simulink model "TRAMI_DCT_AT"  (R2018b)
settings: Solver=FixedStepDiscrete  StartTime=0.0  StopTime=88  FixedStep=10e-3  RelTol=1e-3  EnableMultiTasking=on
undefined symbols (not defined in the file): CONST_AP_GEAR_SUB_NEWTRAL, CONST_AP_IDLE_SPEED_CONT, CONST_AP_LOAD_SFT, CONST_AP_LOAD_SFT_HYS, CONST_CAR_WEIGHT, CONST_CL_NUM, CONST_F_DOWN_SYNCHRO, CONST_F_SYNCHRO, CONST_F_UP_SYNCHRO, CONST_FGR, CONST_I_FlYWHEEL, CONST_INATIA_CLANK, CONST_R_SHIFT_END_CD, CONST_R_SHIFT_END_EG, CONST_R_SHIFT_END_TD, CONST_R_SHIFT_END_UP, CONST_R_SYNCHRO_ENGAGE, CONST_R_TIRE, CONST_RATIO_TQ_REDUCTION, CONST_SKIP_SHIFT_MAX, CONST_SYN_NUM, CONST_T_SFT_END_EN, CONST_T_SFT_END_JUDGE, CONST_T_SFT_END_MAX, CONST_T_SFT_END_MIN, CONST_T_SHIFT_WAIT, CONST_T_TQ_PHASE_CD, CONST_T_TQ_PHASE_ND, CONST_T_TQ_PHASE_NR, CONST_T_TQ_PHASE_TD, CONST_T_TQ_PHASE_UP, CONST_TQ_CREEP_CONT, CONST_TQ_ENGAGE_CL_MARGIN, CONST_TQ_ENGAGE_CL_MIN, CONST_TQ_INATIA_TD_SHIFT, CONST_TQ_LOAD_SFT, CONST_TQ_LOAD_SFT_HYS, CONST_TQ_ND_ENGAGE, CONST_TQ_NR_ENGAGE, CONST_TQ_TQPHASE_MIN, CONST_V_IDLE_SPEED_CONT, Eng, FALSE, GrNP, GrRev, LoopTime, MAT_CL_ENGAGE, MAT_CL_SHARE_RATE, MAT_I_ACTUATOR, MAT_SYNCHRO_COM, MAT_T_GEAR_SUB_NEWTRAL, MAT_TRANS_MGR, MaxCL, Nm, PI, Shift_CD, Shift_ND, Shift_NR, Shift_TD, Shift_Up ... (+168)
libraries: simulink x26
(part 4 of 6)

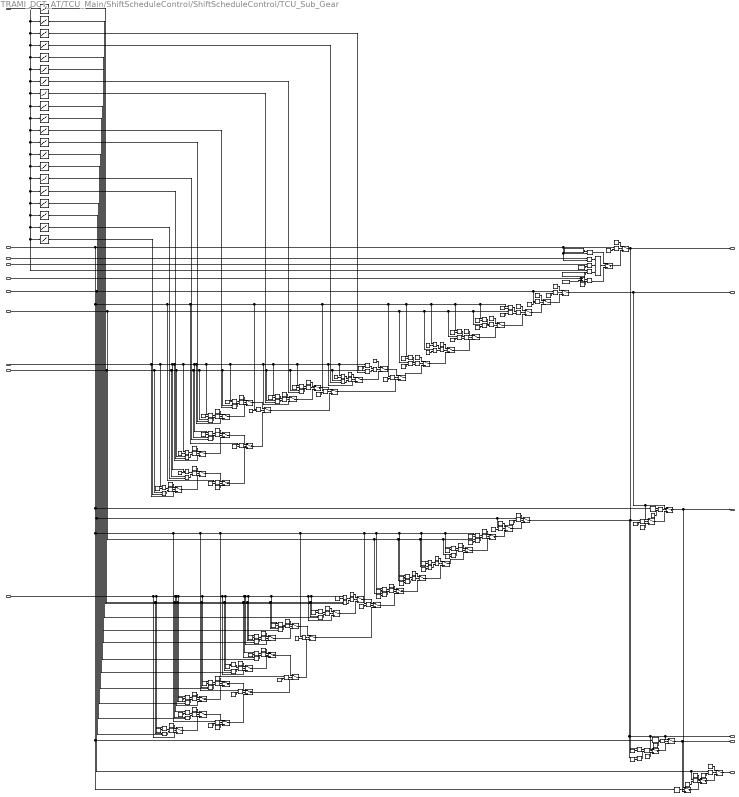
== system TRAMI_DCT_AT/TCU_Main/ShiftScheduleControl/ShiftScheduleControl/TCU_Sub_Gear ==
  accel_position : Inport  OutDataTypeStr=single
      settings: AttributesFormatString=アクセル開度[%]
  v_vehicle : Inport  Port=2  OutDataTypeStr=single
      settings: AttributesFormatString=車速[km/h]
  gear_target : Inport  Port=3  OutDataTypeStr=int16
      settings: AttributesFormatString=目標ギヤ段[-]
  gear_target_old : Inport  Port=4  OutDataTypeStr=int16
      settings: AttributesFormatString=前回の目標ギヤ段[-]
  gear_before_shift : Inport  Port=5  OutDataTypeStr=int16
      settings: AttributesFormatString=変速前ギヤ段[-]
  shifter_position : Inport  Port=6  OutDataTypeStr=int16
      settings: AttributesFormatString=|
      | シフター位置
      |  (Rev=-1; N=0 ; D=1)
      | [-]
  flag_shift : Inport  Port=7  OutDataTypeStr=boolean
      settings: AttributesFormatString=シフトフラグ[-]
  t_neutral_old : Inport  Port=8  OutDataTypeStr=single
      settings: AttributesFormatString=前回のニュートラル移行時間[ms]
  gear_sub1_tmp_old : Inport  Port=9  OutDataTypeStr=int16
      settings: AttributesFormatString=前回の待機ギヤ段（奇数軸）用中間データ[-]
  gear_sub2_tmp_old : Inport  Port=10  OutDataTypeStr=int16
      settings: AttributesFormatString=前回の待機ギヤ段（偶数軸）用中間データ[-]
  Add : Sum  Inputs=+-  OutDataTypeStr=single
  Bitwise Operator : simulink/Logic and Bit Operations/Bitwise Operator  logicop=AND  UseBitMask=on  BitMask=hex2dec('01')  BitMaskRealWorld=Stored Integer
  Bitwise Operator1 : simulink/Logic and Bit Operations/Bitwise Operator  logicop=AND  UseBitMask=on  BitMask=hex2dec('01')  BitMaskRealWorld=Stored Integer
  Bitwise Operator2 : simulink/Logic and Bit Operations/Bitwise Operator  logicop=AND  UseBitMask=on  BitMask=hex2dec('01')  BitMaskRealWorld=Stored Integer
  Constant : Constant  Value=GrRev  OutDataTypeStr=int16
  Constant1 : Constant  Value=0.0  OutDataTypeStr=single
  Constant10 : Constant  Value=0.0  OutDataTypeStr=single
  Constant{46,61,65,70,96..97,100..101} (8 alike) : Constant  Value=5  OutDataTypeStr=int16
  Constant{6,12..14,31,33,36,64,67,69,81,85,92,99,102,107,112} (17 alike) : Constant  Value=0  OutDataTypeStr=int16
  Constant{53,71..73,103..106} (8 alike) : Constant  Value=3  OutDataTypeStr=int16
  Constant{60,66,74..76,108..109} (7 alike) : Constant  OutDataTypeStr=int16
  Constant11 : Constant  Value=-1  OutDataTypeStr=int16
  Constant{27..29,57,59,62..63,110} (8 alike) : Constant  Value=2  OutDataTypeStr=int16
  Constant{15..17,34..35,77,79,88} (8 alike) : Constant  Value=10  OutDataTypeStr=int16
  Constant{18..20,37..38,41..42,82,84} (9 alike) : Constant  Value=8  OutDataTypeStr=int16
  Constant2 : Constant  Value=TRUE  OutDataTypeStr=boolean
  Constant{21..23,43,45,48..49,91} (8 alike) : Constant  Value=6  OutDataTypeStr=int16
  Constant{24..26,50,52,55..56,98} (8 alike) : Constant  Value=4  OutDataTypeStr=int16
  Constant{30,40,44,47,83,86..87} (7 alike) : Constant  Value=9  OutDataTypeStr=int16
  Constant{39,51,54,58,89..90,93..94} (8 alike) : Constant  Value=7  OutDataTypeStr=int16
  Constant5 : Constant  Value=-1  OutDataTypeStr=int16
  Constant68 : Constant  Value=0.0  OutDataTypeStr=single
  Constant7 : Constant  Value=CONST_AP_GEAR_SUB_NEWTRAL  OutDataTypeStr=int16
  Constant8 : Constant  Value=MAT_T_GEAR_SUB_NEWTRAL  OutDataTypeStr=int16
  Constant80 : Constant  Value=11  OutDataTypeStr=int16
  Constant9 : Constant  Value=LoopTime  OutDataTypeStr=single
  Constant95 : Constant  Value=-1  OutDataTypeStr=int16
  Logical Operator : Logic  Operator=OR  Inputs=3  AllPortsSameDT=off  OutDataTypeStr=boolean
  Logical Operator{1..15,17..31} (30 alike) : Logic  Operator=OR  AllPortsSameDT=off  OutDataTypeStr=boolean
  Logical Operator33 : Logic  AllPortsSameDT=off  OutDataTypeStr=boolean
  MinMax : MinMax  Function=max  Inputs=2  OutDataTypeStr=single
  Relational Operator{,2,6..18,23,28,33,38,43,45..57,62,67,72,77,85..86} (39 alike) : RelationalOperator  Operator===  OutDataTypeStr=boolean  RndMeth=Nearest
  Relational Operator1 : RelationalOperator  Operator=~=  OutDataTypeStr=boolean  RndMeth=Nearest
  Relational Operator{19,24,29,34,39,44,58,63,68,73,78,82..83} (13 alike) : RelationalOperator  Operator=>  OutDataTypeStr=boolean  RndMeth=Nearest
  Relational Operator{20,25,30,35,40,59,64,69,74,79} (10 alike) : RelationalOperator  OutDataTypeStr=boolean  RndMeth=Nearest
  Relational Operator{5,21..22,26..27,31..32,36..37,41..42,60..61,65..66,70..71,75..76,80..81} (21 alike) : RelationalOperator  Operator=<  OutDataTypeStr=boolean  RndMeth=Nearest
  Relational Operator84 : RelationalOperator  Operator=<=  OutDataTypeStr=boolean  RndMeth=Nearest
  Selector : Selector  IndexMode=Zero-based  InputPortWidth=11  IndexOptions=Index vector (port)  Indices=[1 3]  OutputSizes=1
  Switch : Switch  Criteria=u2 > Threshold  OutDataTypeStr=single
  Switch1 : Switch  Criteria=u2 > Threshold  OutDataTypeStr=single
  Switch{2..52} (51 alike) : Switch  Criteria=u2 > Threshold  OutDataTypeStr=int16
  Table_search_2D1 : Lookup_n-D  NumberOfTableDimensions=1  BreakpointsForDimension1=T2D_V_SGR_10D_X  Table=T2D_V_SGR_10D_Y  TableDataTypeStr=single  ExtrapMethod=Clip  UseLastTableValue=on  InternalRulePriority=Speed  OutDataTypeStr=single  RndMeth=Simplest  InputSameDT=on
      settings: AttributesFormatString=|
      | tbl = %<Table>
      | axis = %<BreakpointsForDimension1>
  Table_search_2D10 : Lookup_n-D  NumberOfTableDimensions=1  BreakpointsForDimension1=T2D_V_SGR_8D_X  Table=T2D_V_SGR_8D_Y  TableDataTypeStr=single  ExtrapMethod=Clip  UseLastTableValue=on  InternalRulePriority=Speed  OutDataTypeStr=single  RndMeth=Simplest  InputSameDT=on
      settings: AttributesFormatString=|
      | tbl = %<Table>
      | axis = %<BreakpointsForDimension1>
  Table_search_2D11 : Lookup_n-D  NumberOfTableDimensions=1  BreakpointsForDimension1=T2D_V_SGR_5D_X  Table=T2D_V_SGR_5D_Y  TableDataTypeStr=single  ExtrapMethod=Clip  UseLastTableValue=on  InternalRulePriority=Speed  OutDataTypeStr=single  RndMeth=Simplest  InputSameDT=on
      settings: AttributesFormatString=|
      | tbl = %<Table>
      | axis = %<BreakpointsForDimension1>
  Table_search_2D12 : Lookup_n-D  NumberOfTableDimensions=1  BreakpointsForDimension1=T2D_V_SGR_3D_X  Table=T2D_V_SGR_3D_Y  TableDataTypeStr=single  ExtrapMethod=Clip  UseLastTableValue=on  InternalRulePriority=Speed  OutDataTypeStr=single  RndMeth=Simplest  InputSameDT=on
      settings: AttributesFormatString=|
      | tbl = %<Table>
      | axis = %<BreakpointsForDimension1>
  Table_search_2D13 : Lookup_n-D  NumberOfTableDimensions=1  BreakpointsForDimension1=T2D_V_SGR_4U_X  Table=T2D_V_SGR_4U_Y  TableDataTypeStr=single  ExtrapMethod=Clip  UseLastTableValue=on  InternalRulePriority=Speed  OutDataTypeStr=single  RndMeth=Simplest  InputSameDT=on
      settings: AttributesFormatString=|
      | tbl = %<Table>
      | axis = %<BreakpointsForDimension1>
  Table_search_2D14 : Lookup_n-D  NumberOfTableDimensions=1  BreakpointsForDimension1=T2D_V_SGR_4D_X  Table=T2D_V_SGR_4D_Y  TableDataTypeStr=single  ExtrapMethod=Clip  UseLastTableValue=on  InternalRulePriority=Speed  OutDataTypeStr=single  RndMeth=Simplest  InputSameDT=on
      settings: AttributesFormatString=|
      | tbl = %<Table>
      | axis = %<BreakpointsForDimension1>
  Table_search_2D15 : Lookup_n-D  NumberOfTableDimensions=1  BreakpointsForDimension1=T2D_V_SGR_3U_X  Table=T2D_V_SGR_3U_Y  TableDataTypeStr=single  ExtrapMethod=Clip  UseLastTableValue=on  InternalRulePriority=Speed  OutDataTypeStr=single  RndMeth=Simplest  InputSameDT=on
      settings: AttributesFormatString=|
      | tbl = %<Table>
      | axis = %<BreakpointsForDimension1>
  Table_search_2D16 : Lookup_n-D  NumberOfTableDimensions=1  BreakpointsForDimension1=T2D_V_SGR_2U_X  Table=T2D_V_SGR_2U_Y  TableDataTypeStr=single  ExtrapMethod=Clip  UseLastTableValue=on  InternalRulePriority=Speed  OutDataTypeStr=single  RndMeth=Simplest  InputSameDT=on
      settings: AttributesFormatString=|
      | tbl = %<Table>
      | axis = %<BreakpointsForDimension1>
  Table_search_2D17 : Lookup_n-D  NumberOfTableDimensions=1  BreakpointsForDimension1=T2D_V_SGR_5U_X  Table=T2D_V_SGR_5U_Y  TableDataTypeStr=single  ExtrapMethod=Clip  UseLastTableValue=on  InternalRulePriority=Speed  OutDataTypeStr=single  RndMeth=Simplest  InputSameDT=on
      settings: AttributesFormatString=|
      | tbl = %<Table>
      | axis = %<BreakpointsForDimension1>
  Table_search_2D18 : Lookup_n-D  NumberOfTableDimensions=1  BreakpointsForDimension1=T2D_V_SGR_2D_X  Table=T2D_V_SGR_2D_Y  TableDataTypeStr=single  ExtrapMethod=Clip  UseLastTableValue=on  InternalRulePriority=Speed  OutDataTypeStr=single  RndMeth=Simplest  InputSameDT=on
      settings: AttributesFormatString=|
      | tbl = %<Table>
      | axis = %<BreakpointsForDimension1>
  Table_search_2D19 : Lookup_n-D  NumberOfTableDimensions=1  BreakpointsForDimension1=T2D_V_SGR_1U_X  Table=T2D_V_SGR_1U_Y  TableDataTypeStr=single  ExtrapMethod=Clip  UseLastTableValue=on  InternalRulePriority=Speed  OutDataTypeStr=single  RndMeth=Simplest  InputSameDT=on
      settings: AttributesFormatString=|
      | tbl = %<Table>
      | axis = %<BreakpointsForDimension1>
  Table_search_2D2 : Lookup_n-D  NumberOfTableDimensions=1  BreakpointsForDimension1=T2D_V_SGR_9U_X  Table=T2D_V_SGR_9U_Y  TableDataTypeStr=single  ExtrapMethod=Clip  UseLastTableValue=on  InternalRulePriority=Speed  OutDataTypeStr=single  RndMeth=Simplest  InputSameDT=on
      settings: AttributesFormatString=|
      | tbl = %<Table>
      | axis = %<BreakpointsForDimension1>
  Table_search_2D20 : Lookup_n-D  NumberOfTableDimensions=1  BreakpointsForDimension1=T2D_V_SGR_1D_X  Table=T2D_V_SGR_1D_Y  TableDataTypeStr=single  ExtrapMethod=Clip  UseLastTableValue=on  InternalRulePriority=Speed  OutDataTypeStr=single  RndMeth=Simplest  InputSameDT=on
      settings: AttributesFormatString=|
      | tbl = %<Table>
      | axis = %<BreakpointsForDimension1>
  Table_search_2D3 : Lookup_n-D  NumberOfTableDimensions=1  BreakpointsForDimension1=T2D_V_SGR_9D_X  Table=T2D_V_SGR_9D_Y  TableDataTypeStr=single  ExtrapMethod=Clip  UseLastTableValue=on  InternalRulePriority=Speed  OutDataTypeStr=single  RndMeth=Simplest  InputSameDT=on
      settings: AttributesFormatString=|
      | tbl = %<Table>
      | axis = %<BreakpointsForDimension1>
  Table_search_2D4 : Lookup_n-D  NumberOfTableDimensions=1  BreakpointsForDimension1=T2D_V_SGR_8U_X  Table=T2D_V_SGR_8U_Y  TableDataTypeStr=single  ExtrapMethod=Clip  UseLastTableValue=on  InternalRulePriority=Speed  OutDataTypeStr=single  RndMeth=Simplest  InputSameDT=on
      settings: AttributesFormatString=|
      | tbl = %<Table>
      | axis = %<BreakpointsForDimension1>
  Table_search_2D5 : Lookup_n-D  NumberOfTableDimensions=1  BreakpointsForDimension1=T2D_V_SGR_7U_X  Table=T2D_V_SGR_7U_Y  TableDataTypeStr=single  ExtrapMethod=Clip  UseLastTableValue=on  InternalRulePriority=Speed  OutDataTypeStr=single  RndMeth=Simplest  InputSameDT=on
      settings: AttributesFormatString=|
      | tbl = %<Table>
      | axis = %<BreakpointsForDimension1>
  Table_search_2D6 : Lookup_n-D  NumberOfTableDimensions=1  BreakpointsForDimension1=T2D_V_SGR_10U_X  Table=T2D_V_SGR_10U_Y  TableDataTypeStr=single  ExtrapMethod=Clip  UseLastTableValue=on  InternalRulePriority=Speed  OutDataTypeStr=single  RndMeth=Simplest  InputSameDT=on
      settings: AttributesFormatString=|
      | tbl = %<Table>
      | axis = %<BreakpointsForDimension1>
  Table_search_2D7 : Lookup_n-D  NumberOfTableDimensions=1  BreakpointsForDimension1=T2D_V_SGR_7D_X  Table=T2D_V_SGR_7D_Y  TableDataTypeStr=single  ExtrapMethod=Clip  UseLastTableValue=on  InternalRulePriority=Speed  OutDataTypeStr=single  RndMeth=Simplest  InputSameDT=on
      settings: AttributesFormatString=|
      | tbl = %<Table>
      | axis = %<BreakpointsForDimension1>
  Table_search_2D8 : Lookup_n-D  NumberOfTableDimensions=1  BreakpointsForDimension1=T2D_V_SGR_6U_X  Table=T2D_V_SGR_6U_Y  TableDataTypeStr=single  ExtrapMethod=Clip  UseLastTableValue=on  InternalRulePriority=Speed  OutDataTypeStr=single  RndMeth=Simplest  InputSameDT=on
      settings: AttributesFormatString=|
      | tbl = %<Table>
      | axis = %<BreakpointsForDimension1>
  Table_search_2D9 : Lookup_n-D  NumberOfTableDimensions=1  BreakpointsForDimension1=T2D_V_SGR_6D_X  Table=T2D_V_SGR_6D_Y  TableDataTypeStr=single  ExtrapMethod=Clip  UseLastTableValue=on  InternalRulePriority=Speed  OutDataTypeStr=single  RndMeth=Simplest  InputSameDT=on
      settings: AttributesFormatString=|
      | tbl = %<Table>
      | axis = %<BreakpointsForDimension1>
  gear_sub : Outport  OutDataTypeStr=int16  PortDimensions=1
      settings: AttributesFormatString=待機ギヤ段[-]
  gear_sub1 : Outport  Port=2  OutDataTypeStr=int16  PortDimensions=1
      settings: AttributesFormatString=待機ギヤ段（奇数軸）
  gear_sub2 : Outport  Port=3  OutDataTypeStr=int16  PortDimensions=1
      settings: AttributesFormatString=待機ギヤ段（偶数軸）[-]
  t_neutral : Outport  Port=4  OutDataTypeStr=single  PortDimensions=1
      settings: AttributesFormatString=ニュートラル移行時間[ms]
  gear_sub1_tmp : Outport  Port=5  OutDataTypeStr=int16  PortDimensions=1
      settings: AttributesFormatString=待機ギヤ段（奇数軸）用中間データ[-]
  gear_sub2_tmp : Outport  Port=6  OutDataTypeStr=int16  PortDimensions=1
      settings: AttributesFormatString=待機ギヤ段（偶数軸）用中間データ[-]
  wires:
  accel_position/1 -> Table_search_2D5/1, Table_search_2D20/1, Relational Operator5/1, Table_search_2D19/1, Table_search_2D18/1, Table_search_2D16/1, Table_search_2D12/1, Table_search_2D15/1, Table_search_2D14/1, Table_search_2D13/1, Table_search_2D11/1, Table_search_2D17/1, Table_search_2D9/1, Table_search_2D8/1, Table_search_2D7/1, Table_search_2D10/1, Table_search_2D4/1, Table_search_2D3/1, Table_search_2D2/1, Table_search_2D1/1, Table_search_2D6/1  "accel_position"
  Relational Operator/1 -> Switch/2
  Constant1/1 -> Switch/1
  Switch1/1 -> Switch/3
  Switch/1 -> t_neutral/1, Relational Operator44/1, Relational Operator83/1  "t_neutral"
  gear_target_old/1 -> Relational Operator1/1  "gear_target_old"
  flag_shift/1 -> Relational Operator2/1  "flag_shift"
  Constant/1 -> Relational Operator/2
  Constant2/1 -> Relational Operator2/2
  gear_sub1_tmp_old/1 -> Relational Operator68/1, Relational Operator58/1, Relational Operator60/1, Switch35/3, Relational Operator63/1, Relational Operator65/1, Switch38/3, Relational Operator70/1, Switch41/3, Relational Operator73/1, Relational Operator75/1, Switch44/3, Relational Operator78/1, Relational Operator80/1, Switch47/3
  Relational Operator1/1 -> Logical Operator/1
  Relational Operator2/1 -> Logical Operator/2
  Constant7/1 -> Relational Operator5/2
  Relational Operator5/1 -> Logical Operator/3
  Logical Operator/1 -> Switch1/2
  Selector/1 -> Switch1/1
  Constant8/1 -> Selector/1
  MinMax/1 -> Switch1/3
  Add/1 -> MinMax/1
  Constant9/1 -> Add/2
  Constant10/1 -> MinMax/2
  t_neutral_old/1 -> Add/1
  Relational Operator6/1 -> Switch2/2
  Constant11/1 -> Relational Operator6/2
  Constant12/1 -> Switch2/1
  Switch3/1 -> Switch2/3
  Relational Operator7/1 -> Switch3/2
  Constant13/1 -> Relational Operator7/2
  Constant14/1 -> Switch3/1
  Switch4/1 -> Switch3/3
  Logical Operator1/1 -> Switch4/2
  Constant15/1 -> Switch4/1
  Relational Operator9/1 -> Logical Operator1/2
  Relational Operator8/1 -> Logical Operator1/1
  Constant16/1 -> Relational Operator8/2
  Constant17/1 -> Relational Operator9/2
  Switch5/1 -> Switch4/3
  Switch6/1 -> Switch5/3
  Constant20/1 -> Relational Operator11/2
  Constant19/1 -> Relational Operator10/2
  Relational Operator10/1 -> Logical Operator2/1
  Relational Operator11/1 -> Logical Operator2/2
  Constant18/1 -> Switch5/1
  Logical Operator2/1 -> Switch5/2
  Logical Operator3/1 -> Switch6/2
  Constant21/1 -> Switch6/1
  Relational Operator13/1 -> Logical Operator3/2
  Relational Operator12/1 -> Logical Operator3/1
  Constant22/1 -> Relational Operator12/2
  Constant23/1 -> Relational Operator13/2
  Switch7/1 -> Switch6/3
  Switch8/1 -> Switch7/3
  Constant26/1 -> Relational Operator15/2
  Constant25/1 -> Relational Operator14/2
  Relational Operator14/1 -> Logical Operator4/1
  Relational Operator15/1 -> Logical Operator4/2
  Constant24/1 -> Switch7/1
  Logical Operator4/1 -> Switch7/2
  Logical Operator5/1 -> Switch8/2
  Constant27/1 -> Switch8/1
  Relational Operator17/1 -> Logical Operator5/2
  Relational Operator16/1 -> Logical Operator5/1
  Constant28/1 -> Relational Operator16/2
  Constant29/1 -> Relational Operator17/2
  Switch9/1 -> Switch8/3
  Relational Operator18/1 -> Switch9/2
  Constant30/1 -> Relational Operator18/2
  Switch10/1 -> Switch9/1
  gear_sub2_tmp_old/1 -> Relational Operator41/1, Relational Operator39/1, Relational Operator36/1, Relational Operator34/1, Relational Operator31/1, Relational Operator29/1, Relational Operator24/1, Relational Operator19/1, Relational Operator21/1, Switch11/3, Relational Operator26/1, Switch14/3, Switch17/3, Switch20/3, Switch23/3  "gear_sub2_tmp"
  Constant34/1 -> Relational Operator19/2
  Logical Operator6/1 -> Switch10/2
  Relational Operator19/1 -> Logical Operator6/1
  Relational Operator20/1 -> Logical Operator6/2
  Table_search_2D2/1 -> Relational Operator20/2  "ans"
  Constant35/1 -> Switch10/1
  Switch11/1 -> Switch10/3
  Constant38/1 -> Switch11/1
  Table_search_2D3/1 -> Relational Operator22/2  "ans"
  Relational Operator22/1 -> Logical Operator7/2
  Relational Operator21/1 -> Logical Operator7/1
  Logical Operator7/1 -> Switch11/2
  Constant37/1 -> Relational Operator21/2
  Switch2/1 -> gear_sub2_tmp/1, Switch25/1, Switch24/1  "gear_sub2_tmp"
  Relational Operator23/1 -> Switch12/2
  Constant39/1 -> Relational Operator23/2
  Switch13/1 -> Switch12/1
  Logical Operator8/1 -> Switch13/2
  Relational Operator24/1 -> Logical Operator8/1
  Constant41/1 -> Relational Operator24/2
  Relational Operator25/1 -> Logical Operator8/2
  Table_search_2D5/1 -> Relational Operator25/2  "ans"
  Constant42/1 -> Switch13/1
  Switch14/1 -> Switch13/3
  Relational Operator27/1 -> Logical Operator9/2
  Relational Operator26/1 -> Logical Operator9/1
  Logical Operator9/1 -> Switch14/2
  Constant43/1 -> Switch14/1
  Constant45/1 -> Relational Operator26/2
  Table_search_2D7/1 -> Relational Operator27/2  "v_shift_sub_7dans"
  Switch15/1 -> Switch12/3
  Switch18/1 -> Switch15/3
  Table_search_2D11/1 -> Relational Operator32/2  "v_shift_sub_7dans"
  Constant52/1 -> Relational Operator31/2
  Constant50/1 -> Switch17/1
  Logical Operator11/1 -> Switch17/2
  Relational Operator31/1 -> Logical Operator11/1
  Relational Operator32/1 -> Logical Operator11/2
  Switch17/1 -> Switch16/3
  Constant49/1 -> Switch16/1
  Table_search_2D17/1 -> Relational Operator30/2  "ans"
  Relational Operator30/1 -> Logical Operator10/2
  Constant48/1 -> Relational Operator29/2
  Relational Operator29/1 -> Logical Operator10/1
  Logical Operator10/1 -> Switch16/2
  Switch16/1 -> Switch15/1
  Constant46/1 -> Relational Operator28/2
  Relational Operator28/1 -> Switch15/2
  Table_search_2D15/1 -> Relational Operator35/2  "v_vehicle"
  Relational Operator33/1 -> Switch18/2
  Constant53/1 -> Relational Operator33/2
  Switch19/1 -> Switch18/1
  Logical Operator12/1 -> Switch19/2
  Relational Operator34/1 -> Logical Operator12/1
  Constant55/1 -> Relational Operator34/2
  Relational Operator35/1 -> Logical Operator12/2
  Constant56/1 -> Switch19/1
  Switch20/1 -> Switch19/3
  Relational Operator37/1 -> Logical Operator13/2
  Relational Operator36/1 -> Logical Operator13/1
  Logical Operator13/1 -> Switch20/2
  Constant57/1 -> Switch20/1
  Constant59/1 -> Relational Operator36/2
  Table_search_2D12/1 -> Relational Operator37/2  "v_shift_sub_7dans"
  Switch21/1 -> Switch18/3
  Table_search_2D20/1 -> Relational Operator42/2  "v_shift_sub_7dans"
  Constant66/1 -> Relational Operator41/2
  Constant64/1 -> Switch23/1
  Logical Operator15/1 -> Switch23/2
  Relational Operator41/1 -> Logical Operator15/1
  Relational Operator42/1 -> Logical Operator15/2
  Switch23/1 -> Switch22/3
  Constant63/1 -> Switch22/1
  Relational Operator40/1 -> Logical Operator14/2
  Constant62/1 -> Relational Operator39/2
  Relational Operator39/1 -> Logical Operator14/1
  Logical Operator14/1 -> Switch22/2
  Switch22/1 -> Switch21/1
  Constant60/1 -> Relational Operator38/2
  Relational Operator38/1 -> Switch21/2
  Table_search_2D19/1 -> Relational Operator40/2  "v_vehicle"
  Bitwise Operator/1 -> Relational Operator43/1
  Constant67/1 -> Relational Operator43/2
  Relational Operator43/1 -> Switch24/2
  Switch25/1 -> Switch24/3
  Relational Operator44/1 -> Switch25/2
  Constant68/1 -> Relational Operator44/2
  Constant69/1 -> Switch25/3
  Constant5/1 -> Relational Operator45/2
  Relational Operator45/1 -> Switch26/2
  Switch27/1 -> Switch26/3
  Constant6/1 -> Switch26/1
  Constant36/1 -> Switch27/1
  Switch28/1 -> Switch27/3
  Relational Operator46/1 -> Switch27/2
  Constant33/1 -> Relational Operator46/2
  Switch26/1 -> Switch48/1, gear_sub1_tmp/1, Switch49/1, Relational Operator84/1  "gear_sub1_tmp"
  Constant40/1 -> Relational Operator47/2
  Relational Operator47/1 -> Logical Operator17/1
  Relational Operator48/1 -> Logical Operator17/2
  Constant44/1 -> Relational Operator48/2
  Logical Operator17/1 -> Switch28/2
  Constant47/1 -> Switch28/1
  Switch29/1 -> Switch28/3
  Logical Operator18/1 -> Switch29/2
  Constant58/1 -> Switch29/1
  Switch30/1 -> Switch29/3
  Relational Operator49/1 -> Logical Operator18/1
  Constant51/1 -> Relational Operator49/2
  Relational Operator50/1 -> Logical Operator18/2
  Constant54/1 -> Relational Operator50/2
  Constant65/1 -> Relational Operator52/2
  Relational Operator52/1 -> Logical Operator19/2
  Constant61/1 -> Relational Operator51/2
  Relational Operator51/1 -> Logical Operator19/1
  Switch31/1 -> Switch30/3
  Constant70/1 -> Switch30/1
  Logical Operator19/1 -> Switch30/2
  Logical Operator20/1 -> Switch31/2
  Constant73/1 -> Switch31/1
  Switch32/1 -> Switch31/3
  Relational Operator53/1 -> Logical Operator20/1
  Constant71/1 -> Relational Operator53/2
  Relational Operator54/1 -> Logical Operator20/2
  Constant72/1 -> Relational Operator54/2
  Constant75/1 -> Relational Operator56/2
  Relational Operator56/1 -> Logical Operator21/2
  Constant74/1 -> Relational Operator55/2
  Relational Operator55/1 -> Logical Operator21/1
  Switch33/1 -> Switch32/3
  Constant76/1 -> Switch32/1
  Logical Operator21/1 -> Switch32/2
  gear_before_shift/1 -> Relational Operator17/1, Relational Operator15/1, Relational Operator13/1, Relational Operator11/1, Relational Operator9/1, Relational Operator54/1, Relational Operator50/1, Relational Operator48/1, Relational Operator52/1, Relational Operator56/1  "gear_before_shift"
  Relational Operator57/1 -> Switch33/2
  Constant77/1 -> Relational Operator57/2
  Relational Operator58/1 -> Logical Operator22/1
  Constant79/1 -> Relational Operator58/2
  Relational Operator59/1 -> Logical Operator22/2
  Table_search_2D6/1 -> Relational Operator59/2  "ans"
  Switch34/1 -> Switch33/1
  Logical Operator22/1 -> Switch34/2
  Constant80/1 -> Switch34/1
  Switch36/1 -> Switch33/3
  Constant83/1 -> Switch35/1
  Logical Operator23/1 -> Switch35/2
  Table_search_2D1/1 -> Relational Operator61/2  "ans"
  Relational Operator61/1 -> Logical Operator23/2
  Constant82/1 -> Relational Operator60/2
  Relational Operator60/1 -> Logical Operator23/1
  Switch35/1 -> Switch34/3
  Switch38/1 -> Switch37/3
  Relational Operator65/1 -> Logical Operator25/1
  Constant89/1 -> Relational Operator65/2
  Relational Operator66/1 -> Logical Operator25/2
  Table_search_2D10/1 -> Relational Operator66/2  "ans"
  Logical Operator25/1 -> Switch38/2
  Constant90/1 -> Switch38/1
  Switch39/1 -> Switch36/3
  Constant87/1 -> Switch37/1
  Logical Operator24/1 -> Switch37/2
  Switch37/1 -> Switch36/1
  Table_search_2D4/1 -> Relational Operator64/2  "ans"
  Relational Operator64/1 -> Logical Operator24/2
  Constant86/1 -> Relational Operator63/2
  Relational Operator63/1 -> Logical Operator24/1
  Constant84/1 -> Relational Operator62/2
  Relational Operator62/1 -> Switch36/2
  Relational Operator67/1 -> Switch39/2
  Constant91/1 -> Relational Operator67/2
  Relational Operator68/1 -> Logical Operator26/1
  Constant93/1 -> Relational Operator68/2
  Relational Operator69/1 -> Logical Operator26/2
  Table_search_2D8/1 -> Relational Operator69/2  "ans"
  Switch40/1 -> Switch39/1
  Logical Operator26/1 -> Switch40/2
  Constant94/1 -> Switch40/1
  Switch42/1 -> Switch39/3
  Constant97/1 -> Switch41/1
  Logical Operator27/1 -> Switch41/2
  Table_search_2D9/1 -> Relational Operator71/2  "ans"
  Relational Operator71/1 -> Logical Operator27/2
  Constant96/1 -> Relational Operator70/2
  Relational Operator70/1 -> Logical Operator27/1
  Switch41/1 -> Switch40/3
  Switch44/1 -> Switch43/3
  Relational Operator75/1 -> Logical Operator29/1
  Constant103/1 -> Relational Operator75/2
  Relational Operator76/1 -> Logical Operator29/2
  Table_search_2D14/1 -> Relational Operator76/2  "ans"
  Logical Operator29/1 -> Switch44/2
  Constant104/1 -> Switch44/1
  Switch45/1 -> Switch42/3
  Constant101/1 -> Switch43/1
  Logical Operator28/1 -> Switch43/2
  Switch43/1 -> Switch42/1
  Table_search_2D13/1 -> Relational Operator74/2  "ans"
  Relational Operator74/1 -> Logical Operator28/2
  Constant100/1 -> Relational Operator73/2
  Relational Operator73/1 -> Logical Operator28/1
  Constant98/1 -> Relational Operator72/2
  Relational Operator72/1 -> Switch42/2
  v_vehicle/1 -> Relational Operator40/1, Relational Operator37/1, Relational Operator35/1, Relational Operator32/1, Relational Operator30/1, Relational Operator27/1, Relational Operator22/1, Relational Operator20/1, Relational Operator25/1, Relational Operator42/1, Relational Operator81/1, Relational Operator79/1, Relational Operator76/1, Relational Operator74/1, Relational Operator71/1, Relational Operator69/1, Relational Operator66/1, Relational Operator61/1, Relational Operator59/1, Relational Operator64/1  "v_vehicle"
  Relational Operator77/1 -> Switch45/2
  Constant110/1 -> Relational Operator77/2
  Relational Operator78/1 -> Logical Operator30/1
  Constant105/1 -> Relational Operator78/2
  Relational Operator79/1 -> Logical Operator30/2
  Table_search_2D16/1 -> Relational Operator79/2  "ans"
  Switch46/1 -> Switch45/1
  Logical Operator30/1 -> Switch46/2
  Constant106/1 -> Switch46/1
  Constant112/1 -> Switch45/3
  Constant109/1 -> Switch47/1
  Logical Operator31/1 -> Switch47/2
  Table_search_2D18/1 -> Relational Operator81/2  "ans"
  Relational Operator81/1 -> Logical Operator31/2
  Constant108/1 -> Relational Operator80/2
  Relational Operator80/1 -> Logical Operator31/1
  Switch47/1 -> Switch46/3
  gear_target/1 -> Relational Operator1/2, Selector/2, Relational Operator/1, Relational Operator8/1, Relational Operator10/1, Relational Operator12/1, Relational Operator14/1, Relational Operator16/1, Relational Operator18/1, Relational Operator23/1, Relational Operator28/1, Relational Operator33/1, Relational Operator38/1, Bitwise Operator/1, Relational Operator77/1, Relational Operator47/1, Relational Operator49/1, Relational Operator51/1, Relational Operator53/1, Relational Operator55/1, Relational Operator57/1, Relational Operator62/1, Relational Operator67/1, Relational Operator72/1, Bitwise Operator1/1, Bitwise Operator2/1
  Bitwise Operator1/1 -> Relational Operator82/1
  Constant81/1 -> Relational Operator82/2
  Relational Operator82/1 -> Switch48/2
  Switch48/1 -> gear_sub1/1, Switch52/3  "gear_sub1"
  Constant85/1 -> Relational Operator83/2
  Relational Operator83/1 -> Logical Operator33/1
  Relational Operator84/1 -> Logical Operator33/2
  Constant88/1 -> Relational Operator84/2
  Logical Operator33/1 -> Switch49/2
  Switch49/1 -> Switch48/3  "gear_sub1"
  Constant92/1 -> Switch49/3
  Relational Operator85/1 -> Switch50/2
  Constant102/1 -> Switch50/1
  Switch51/1 -> Switch50/3
  shifter_position/1 -> Relational Operator6/1, Relational Operator7/1, Relational Operator46/1, Relational Operator45/1, Relational Operator86/1, Relational Operator85/1  "shifter_position"
  Constant95/1 -> Relational Operator85/2
  Constant99/1 -> Relational Operator86/2
  Switch52/1 -> Switch51/3
  Constant107/1 -> Switch51/1
  Relational Operator86/1 -> Switch51/2
  Bitwise Operator2/1 -> Switch52/2
  Switch50/1 -> gear_sub/1  "gear_sub"
  Switch24/1 -> gear_sub2/1, Switch52/1  "gear_sub2"
  Constant31/1 -> Switch21/3
  Switch12/1 -> Switch9/3

== system TRAMI_DCT_AT/TCU_Main/ShiftScheduleControl/ShiftScheduleControl/TCU_Tsp_Each_Gear ==
  r_gearbox_output : Inport  OutDataTypeStr=single
      settings: AttributesFormatString=GearBox出力回転[rpm]
  Gain : Gain  Gain=MAT_TRANS_MGR  OutDataTypeStr=single
  r_gb_input_each_gear : Outport  OutDataTypeStr=single
      settings: AttributesFormatString=|
      | 各ギヤ段でのGearBox入力回転
      | 配列数12: 左から N, 1st, 2nd, 3rd ,4th ,5th ,6th ,7th, 8th, 9th, 10th, Rev[rpm]
  wires:
  r_gearbox_output/1 -> Gain/1
  Gain/1 -> r_gb_input_each_gear/1  "r_gb_input_each_gear"

== system TRAMI_DCT_AT/TCU_Main/ShiftScheduleControl/ShiftScheduleControl/cUnitDelay1 ==
  <param> : Inport
  Constant13 : Constant  Value=initParam  OutDataTypeStr=int16
  Switch12 : Switch  Criteria=u2 > Threshold
  Unit Delay2 : UnitDelay  InitialCondition=zeros(size(initParam))  SampleTime=-1
  preParam : Outport
  wires:
  <param>/1 -> Unit Delay2/1
  Constant13/1 -> Switch12/1
  [FlagInit] -> Switch12/2
  Switch12/1 -> preParam/1
  Unit Delay2/1 -> Switch12/3

== system TRAMI_DCT_AT/TCU_Main/ShiftScheduleControl/ShiftScheduleControl/cUnitDelay10 ==
  <param> : Inport
  Constant13 : Constant  Value=initParam  OutDataTypeStr=single
  Switch12 : Switch  Criteria=u2 > Threshold
  Unit Delay2 : UnitDelay  InitialCondition=zeros(size(initParam))  SampleTime=-1
  preParam : Outport
  wires:
  Unit Delay2/1 -> Switch12/3
  Switch12/1 -> preParam/1
  [FlagInit] -> Switch12/2
  Constant13/1 -> Switch12/1
  <param>/1 -> Unit Delay2/1

== system TRAMI_DCT_AT/TCU_Main/ShiftScheduleControl/ShiftScheduleControl/cUnitDelay11 ==
  <param> : Inport
  Constant13 : Constant  Value=initParam  OutDataTypeStr=boolean
  Switch12 : Switch  Criteria=u2 > Threshold
  Unit Delay2 : UnitDelay  InitialCondition=zeros(size(initParam))  SampleTime=-1
  preParam : Outport
  wires:
  Unit Delay2/1 -> Switch12/3
  Switch12/1 -> preParam/1
  [FlagInit] -> Switch12/2
  Constant13/1 -> Switch12/1
  <param>/1 -> Unit Delay2/1

== system TRAMI_DCT_AT/TCU_Main/ShiftScheduleControl/ShiftScheduleControl/cUnitDelay12 ==
  <param> : Inport
  Constant13 : Constant  Value=initParam  OutDataTypeStr=single
  Switch12 : Switch  Criteria=u2 > Threshold
  Unit Delay2 : UnitDelay  InitialCondition=zeros(size(initParam))  SampleTime=-1
  preParam : Outport
  wires:
  <param>/1 -> Unit Delay2/1
  Constant13/1 -> Switch12/1
  [FlagInit] -> Switch12/2
  Switch12/1 -> preParam/1
  Unit Delay2/1 -> Switch12/3

== system TRAMI_DCT_AT/TCU_Main/ShiftScheduleControl/ShiftScheduleControl/cUnitDelay13 ==
  <param> : Inport
  Constant13 : Constant  Value=initParam  OutDataTypeStr=int16
  Switch12 : Switch  Criteria=u2 > Threshold
  Unit Delay2 : UnitDelay  InitialCondition=zeros(size(initParam))  SampleTime=-1
  preParam : Outport  OutDataTypeStr=int16
  wires:
  Unit Delay2/1 -> Switch12/3
  Switch12/1 -> preParam/1
  [FlagInit] -> Switch12/2
  Constant13/1 -> Switch12/1
  <param>/1 -> Unit Delay2/1

== system TRAMI_DCT_AT/TCU_Main/ShiftScheduleControl/ShiftScheduleControl/cUnitDelay14 ==
  <param> : Inport
  Constant13 : Constant  Value=initParam  OutDataTypeStr=single
  Switch12 : Switch  Criteria=u2 > Threshold
  Unit Delay2 : UnitDelay  InitialCondition=zeros(size(initParam))  SampleTime=-1
  preParam : Outport
  wires:
  Unit Delay2/1 -> Switch12/3
  Switch12/1 -> preParam/1
  [FlagInit] -> Switch12/2
  Constant13/1 -> Switch12/1
  <param>/1 -> Unit Delay2/1

== system TRAMI_DCT_AT/TCU_Main/ShiftScheduleControl/ShiftScheduleControl/cUnitDelay15 ==
  <param> : Inport
  Constant13 : Constant  Value=initParam  OutDataTypeStr=int16
  Switch12 : Switch  Criteria=u2 > Threshold
  Unit Delay2 : UnitDelay  InitialCondition=zeros(size(initParam))  SampleTime=-1
  preParam : Outport
  wires:
  <param>/1 -> Unit Delay2/1
  Constant13/1 -> Switch12/1
  [FlagInit] -> Switch12/2
  Switch12/1 -> preParam/1
  Unit Delay2/1 -> Switch12/3

== system TRAMI_DCT_AT/TCU_Main/ShiftScheduleControl/ShiftScheduleControl/cUnitDelay2 ==
  <param> : Inport
  Constant13 : Constant  Value=initParam  OutDataTypeStr=int16
  Switch12 : Switch  Criteria=u2 > Threshold
  Unit Delay2 : UnitDelay  InitialCondition=zeros(size(initParam))  SampleTime=-1
  preParam : Outport
  wires:
  Unit Delay2/1 -> Switch12/3
  Switch12/1 -> preParam/1
  [FlagInit] -> Switch12/2
  Constant13/1 -> Switch12/1
  <param>/1 -> Unit Delay2/1

== system TRAMI_DCT_AT/TCU_Main/ShiftScheduleControl/ShiftScheduleControl/cUnitDelay3 ==
  <param> : Inport
  Constant13 : Constant  Value=initParam  OutDataTypeStr=int16
  Switch12 : Switch  Criteria=u2 > Threshold
  Unit Delay2 : UnitDelay  InitialCondition=zeros(size(initParam))  SampleTime=-1
  preParam : Outport
  wires:
  <param>/1 -> Unit Delay2/1
  Constant13/1 -> Switch12/1
  [FlagInit] -> Switch12/2
  Switch12/1 -> preParam/1
  Unit Delay2/1 -> Switch12/3

== system TRAMI_DCT_AT/TCU_Main/ShiftScheduleControl/ShiftScheduleControl/cUnitDelay4 ==
  <param> : Inport
  Constant13 : Constant  Value=initParam  OutDataTypeStr=boolean
  Switch12 : Switch  Criteria=u2 > Threshold
  Unit Delay2 : UnitDelay  InitialCondition=zeros(size(initParam))  SampleTime=-1
  preParam : Outport
  wires:
  Unit Delay2/1 -> Switch12/3
  Switch12/1 -> preParam/1
  [FlagInit] -> Switch12/2
  Constant13/1 -> Switch12/1
  <param>/1 -> Unit Delay2/1

== system TRAMI_DCT_AT/TCU_Main/ShiftScheduleControl/ShiftScheduleControl/cUnitDelay5 ==
  <param> : Inport
  Constant13 : Constant  Value=initParam  OutDataTypeStr=boolean
  Switch12 : Switch  Criteria=u2 > Threshold  OutDataTypeStr=boolean
  Unit Delay2 : UnitDelay  InitialCondition=zeros(size(initParam))  SampleTime=-1
  preParam : Outport
  wires:
  <param>/1 -> Unit Delay2/1
  Constant13/1 -> Switch12/1
  [FlagInit] -> Switch12/2
  Switch12/1 -> preParam/1
  Unit Delay2/1 -> Switch12/3

== system TRAMI_DCT_AT/TCU_Main/ShiftScheduleControl/ShiftScheduleControl/cUnitDelay6 ==
  <param> : Inport
  Constant13 : Constant  Value=initParam  OutDataTypeStr=boolean
  Switch12 : Switch  Criteria=u2 > Threshold
  Unit Delay2 : UnitDelay  InitialCondition=zeros(size(initParam))  SampleTime=-1
  preParam : Outport
  wires:
  <param>/1 -> Unit Delay2/1
  Constant13/1 -> Switch12/1
  [FlagInit] -> Switch12/2
  Switch12/1 -> preParam/1
  Unit Delay2/1 -> Switch12/3

== system TRAMI_DCT_AT/TCU_Main/ShiftScheduleControl/ShiftScheduleControl/cUnitDelay7 ==
  <param> : Inport
  Constant13 : Constant  Value=initParam  OutDataTypeStr=int16
  Switch12 : Switch  Criteria=u2 > Threshold
  Unit Delay2 : UnitDelay  InitialCondition=zeros(size(initParam))  SampleTime=-1
  preParam : Outport
  wires:
  Unit Delay2/1 -> Switch12/3
  Switch12/1 -> preParam/1
  [FlagInit] -> Switch12/2
  Constant13/1 -> Switch12/1
  <param>/1 -> Unit Delay2/1

== system TRAMI_DCT_AT/TCU_Main/ShiftScheduleControl/ShiftScheduleControl/cUnitDelay8 ==
  <param> : Inport
  Constant13 : Constant  Value=initParam  OutDataTypeStr=int16
  Switch12 : Switch  Criteria=u2 > Threshold
  Unit Delay2 : UnitDelay  InitialCondition=zeros(size(initParam))  SampleTime=-1
  preParam : Outport
  wires:
  <param>/1 -> Unit Delay2/1
  Constant13/1 -> Switch12/1
  [FlagInit] -> Switch12/2
  Switch12/1 -> preParam/1
  Unit Delay2/1 -> Switch12/3

== system TRAMI_DCT_AT/TCU_Main/ShiftScheduleControl/ShiftScheduleControl/cUnitDelay9 ==
  <param> : Inport
  Constant13 : Constant  Value=initParam  OutDataTypeStr=boolean
  Switch12 : Switch  Criteria=u2 > Threshold
  Unit Delay2 : UnitDelay  InitialCondition=zeros(size(initParam))  SampleTime=-1
  preParam : Outport
  wires:
  Unit Delay2/1 -> Switch12/3
  Switch12/1 -> preParam/1
  [FlagInit] -> Switch12/2
  Constant13/1 -> Switch12/1
  <param>/1 -> Unit Delay2/1

== system TRAMI_DCT_AT/TCU_Main/StartingDeviceControl/StartingDeviceControl/TCU_Creep_Control ==
  gear_target : Inport  OutDataTypeStr=int16
      settings: AttributesFormatString=目標ギヤ段[-]
  Compare To Zero : simulink/Logic and Bit Operations/Compare To Zero  relop===  OutDataTypeStr=boolean
  Constant : Constant  Value=0.0  OutDataTypeStr=single
  Constant1 : Constant  Value=CONST_TQ_CREEP_CONT  OutDataTypeStr=single
  Switch1 : Switch  Criteria=u2 ~= 0  OutDataTypeStr=single
  tq_cl_creep_cont : Outport  OutDataTypeStr=single
      settings: AttributesFormatString=クリープ制御のためのクラッチトルク容量[Nm]
  wires:
  gear_target/1 -> Compare To Zero/1
  Compare To Zero/1 -> Switch1/2
  Constant/1 -> Switch1/1
  Constant1/1 -> Switch1/3
  Switch1/1 -> tq_cl_creep_cont/1  "tq_cl_creep_cont"

== system TRAMI_DCT_AT/TCU_Main/StartingDeviceControl/StartingDeviceControl/TCU_Engin_Idle_Control ==
  note: Engineによるアイドル回転制御の実行判定
  <r_engine_idle> : Inport  OutDataTypeStr=single
      settings: AttributesFormatString=エンジンアイドル回転[rpm]
  <accel_position> : Inport  Port=2  OutDataTypeStr=single
      settings: AttributesFormatString=アクセル開度[%]
  <v_vehicle> : Inport  Port=3  OutDataTypeStr=single
      settings: AttributesFormatString=車速[km/h]
  <gear_target> : Inport  Port=4  OutDataTypeStr=int16
      settings: AttributesFormatString=目標ギヤ段[-]
  <r_gb_input_tg_gear> : Inport  Port=5  OutDataTypeStr=single
      settings: AttributesFormatString=|
      | 目標ギヤ段によるGearbox入力回転
      | (GearBox出力回転から演算)[rpm]
  Constant10 : Constant  Value=0  OutDataTypeStr=boolean
  Constant5 : Constant  Value=CONST_AP_IDLE_SPEED_CONT  OutDataTypeStr=single
  Constant9 : Constant  Value=CONST_V_IDLE_SPEED_CONT  OutDataTypeStr=single
  Logical Operator6 : Logic  AllPortsSameDT=off  OutDataTypeStr=boolean
  Logical Operator7 : Logic  Operator=OR  Inputs=3  AllPortsSameDT=off  OutDataTypeStr=boolean
  Relational Operator4 : RelationalOperator  Operator=<  OutDataTypeStr=boolean  RndMeth=Nearest
  Relational Operator6 : RelationalOperator  Operator=<  OutDataTypeStr=boolean  RndMeth=Nearest
  Relational Operator8 : RelationalOperator  Operator=<  OutDataTypeStr=boolean  RndMeth=Nearest
  Relational Operator9 : RelationalOperator  Operator===  OutDataTypeStr=boolean  RndMeth=Nearest
  <flag_engine_idle_control> : Outport  OutDataTypeStr=boolean
      settings: AttributesFormatString=|
      | アイドル回転制御の実行判定フラグ[-]
      | TRUE:エンジンによるアイドル回転制御を実行
      | FALSE:クラッチスリップ制御によるエンジン回転制御を行う
  wires:
  <r_engine_idle>/1 -> Relational Operator4/2  "r_engine_idle"
  Relational Operator4/1 -> Logical Operator6/1
  <accel_position>/1 -> Relational Operator6/1  "accel_position"
  Constant5/1 -> Relational Operator6/2
  Relational Operator6/1 -> Logical Operator6/2
  Logical Operator6/1 -> Logical Operator7/2
  Constant9/1 -> Relational Operator8/2
  Relational Operator8/1 -> Logical Operator7/3
  Constant10/1 -> Relational Operator9/2
  Relational Operator9/1 -> Logical Operator7/1
  Logical Operator7/1 -> <flag_engine_idle_control>/1  "flag_engine_idle_control"
  <r_gb_input_tg_gear>/1 -> Relational Operator4/1  "r_gb_input_tg_gear"
  <gear_target>/1 -> Relational Operator9/1  "gear_target"
  <v_vehicle>/1 -> Relational Operator8/1  "v_vehicle"

== system TRAMI_DCT_AT/TCU_Main/StartingDeviceControl/StartingDeviceControl/TCU_Fluid_Coupling_Torque ==
  r_engine : Inport  OutDataTypeStr=single
      settings: AttributesFormatString=エンジン回転数[rpm]
  r_gearbox_input : Inport  Port=2  OutDataTypeStr=single
      settings: AttributesFormatString=Gearbox input speed[rpm]
  Constant1 : Constant  Value=0.0  OutDataTypeStr=single
  Constant2 : Constant  Value=100.0  OutDataTypeStr=single
  Constant3 : Constant  Value=1000000.0  OutDataTypeStr=single
  Divide : Product  Inputs=*/  OutDataTypeStr=single
  Divide1 : Product  Inputs=**  OutDataTypeStr=single
  Divide2 : Product  Inputs=**  OutDataTypeStr=single
  Divide3 : Product  Inputs=*/  OutDataTypeStr=single
  Divide4 : Product  Inputs=**  OutDataTypeStr=single
  Relational Operator5 : RelationalOperator  Operator=<=  OutDataTypeStr=boolean  RndMeth=Nearest
  Switch1 : Switch  Criteria=u2 ~= 0  OutDataTypeStr=single
  Table_search_2D1 : Lookup_n-D  NumberOfTableDimensions=1  BreakpointsForDimension1=T2D_COUPLING_TQ_RATIO_X  Table=T2D_COUPLING_TQ_RATIO_Y  ExtrapMethod=Clip  UseLastTableValue=on  InternalRulePriority=Speed  OutDataTypeStr=single  RndMeth=Simplest  InputSameDT=on
      settings: AttributesFormatString=|
      | tbl = %<Table>
      | axis = %<BreakpointsForDimension1>
  Table_search_2D8 : Lookup_n-D  NumberOfTableDimensions=1  BreakpointsForDimension1=T2D_COUPLING_CAP_FACT_X  Table=T2D_COUPLING_CAP_FACT_Y  ExtrapMethod=Clip  UseLastTableValue=on  InternalRulePriority=Speed  OutDataTypeStr=single  RndMeth=Simplest  InputSameDT=on
      settings: AttributesFormatString=|
      | tbl = %<Table>
      | axis = %<BreakpointsForDimension1>
  tq_torq_converter_input : Outport  OutDataTypeStr=single
      settings: AttributesFormatString=トルコン流体伝達トルク(入力）[Nm]
  tq_torq_converter_output : Outport  Port=2  OutDataTypeStr=single
      settings: AttributesFormatString=トルコン流体伝達トルク(出力)[Nm]
  spd_ratio_torq_converter : Outport  Port=3  OutDataTypeStr=single
      settings: AttributesFormatString=速度比[-]
  torq_ratio_torq_converter : Outport  Port=4  OutDataTypeStr=single
      settings: AttributesFormatString=トルク比[-]
  cap_factor_torq_converter : Outport  Port=5  OutDataTypeStr=single
      settings: AttributesFormatString=容量係数 [uNm/rpm2]
  wires:
  Relational Operator5/1 -> Switch1/2
  Constant2/1 -> Relational Operator5/2
  r_engine/1 -> Divide2/2, Divide1/2, Divide/2, Relational Operator5/1  "r_engine"
  Constant1/1 -> Switch1/1
  Divide/1 -> Switch1/3
  Switch1/1 -> spd_ratio_torq_converter/1, Table_search_2D8/1, Table_search_2D1/1  "spd_ratio_torq_converter"
  r_gearbox_input/1 -> Divide/1
  Table_search_2D1/1 -> torq_ratio_torq_converter/1, Divide4/2  "torq_ratio_torq_converter"
  Divide1/1 -> Divide2/1
  Divide2/1 -> Divide3/1
  Constant3/1 -> Divide3/2
  Divide3/1 -> tq_torq_converter_input/1, Divide4/1  "tq_torq_converter_input"
  Divide4/1 -> tq_torq_converter_output/1  "tq_torq_converter_output"
  Table_search_2D8/1 -> cap_factor_torq_converter/1, Divide1/1  "cap_factor_torq_converter"
